simulink model "Part_three_homework_eight"  (R2018a)
settings: Solver=VariableStepAuto  StartTime=0.0  StopTime=10  RelTol=1e-3
settings Model: Creator=kr27867  LastModifiedBy=kr27867

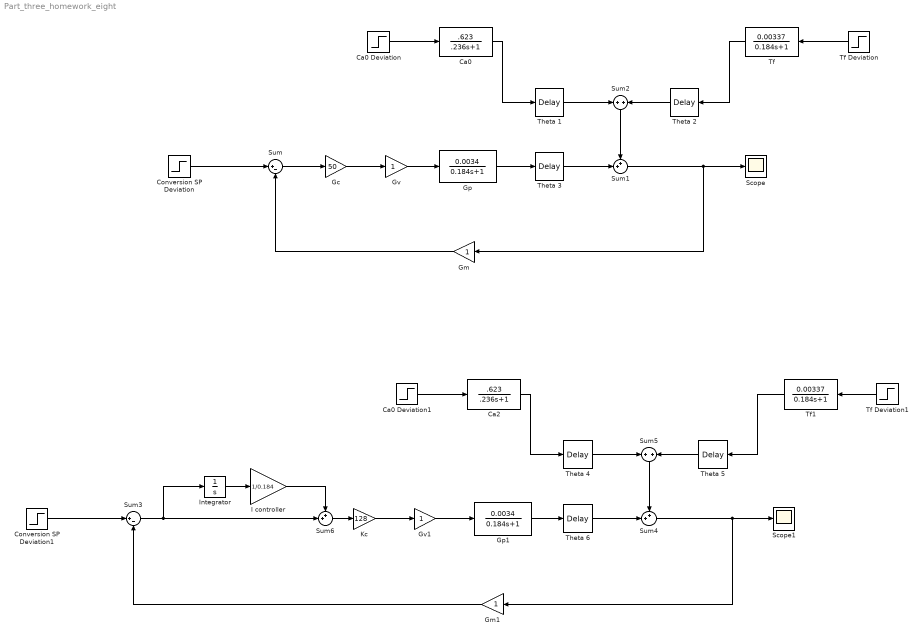
== system Part_three_homework_eight ==
  Ca0 : TransferFcn  Numerator=[.623]  Denominator=[.236 1]
  Ca0 Deviation : Step  Time=0  After=0  SampleTime=0
  Ca0 Deviation1 : Step  Time=0  After=0  SampleTime=0
  Ca2 : TransferFcn  Numerator=[.623]  Denominator=[.236 1]
  Conversion SP Deviation : Step  Before=0.0  After=0  SampleTime=0
  Conversion SP Deviation1 : Step  Before=0.0  After=0  SampleTime=0
  Gc : Gain  Gain=50
  Gm : Gain
  Gm1 : Gain
  Gp : TransferFcn  Numerator=[0.0034]  Denominator=[0.184 1]
  Gp1 : TransferFcn  Numerator=[0.0034]  Denominator=[0.184 1]
  Gv : Gain
  Gv1 : Gain
  I controller : Gain  Gain=1/0.184
  Integrator : Integrator
  Kc : Gain  Gain=128
  Scope : Scope
  Scope1 : Scope
  Sum : Sum  Inputs=|+-
  Sum1 : Sum  Inputs=++|
  Sum2 : Sum  Inputs=+|+
  Sum3 : Sum  Inputs=|+-
  Sum4 : Sum  Inputs=++|
  Sum5 : Sum  Inputs=+|+
  Sum6 : Sum  Inputs=++|
  Tf : TransferFcn  Numerator=[0.00337]  Denominator=[0.184 1]
  Tf Deviation : Step  Time=0  After=-5  SampleTime=0
  Tf Deviation1 : Step  Time=0  After=-5  SampleTime=0
  Tf1 : TransferFcn  Numerator=[0.00337]  Denominator=[0.184 1]
  Theta 1 : TransportDelay  DelayTime=0.267
  Theta 2 : TransportDelay  DelayTime=0.2125
  Theta 3 : TransportDelay  DelayTime=0.212
  Theta 4 : TransportDelay  DelayTime=0.267
  Theta 5 : TransportDelay  DelayTime=0.2125
  Theta 6 : TransportDelay  DelayTime=0.212
  wires:
  Conversion SP Deviation/1 -> Sum/1
  Sum/1 -> Gc/1
  Gc/1 -> Gv/1
  Gp/1 -> Theta 3/1
  Gm/1 -> Sum/2
  Sum1/1 -> Gm/1, Scope/1
  Theta 3/1 -> Sum1/2
  Sum2/1 -> Sum1/1
  Theta 2/1 -> Sum2/2
  Theta 1/1 -> Sum2/1
  Tf/1 -> Theta 2/1
  Ca0/1 -> Theta 1/1
  Tf Deviation/1 -> Tf/1
  Ca0 Deviation/1 -> Ca0/1
  Gv/1 -> Gp/1
  Sum5/1 -> Sum4/1
  Theta 5/1 -> Sum5/2
  Sum4/1 -> Gm1/1, Scope1/1
  Gv1/1 -> Gp1/1
  Tf Deviation1/1 -> Tf1/1
  Conversion SP Deviation1/1 -> Sum3/1
  Ca2/1 -> Theta 4/1
  Kc/1 -> Gv1/1
  Ca0 Deviation1/1 -> Ca2/1
  Gp1/1 -> Theta 6/1
  Theta 6/1 -> Sum4/2
  Gm1/1 -> Sum3/2
  Theta 4/1 -> Sum5/1
  Sum3/1 -> Sum6/2, Integrator/1
  Integrator/1 -> I controller/1
  I controller/1 -> Sum6/1
  Sum6/1 -> Kc/1
  Tf1/1 -> Theta 5/1
